simulink library "optimum_ul"  (R2018a)
settings: Solver=VariableStepAuto  StartTime=0.0  StopTime=10.0  RelTol=1e-3
settings Model: Creator=mitch  LastModifiedBy=mitch

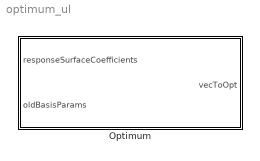
== system optimum_ul ==
  Optimum : Subsystem

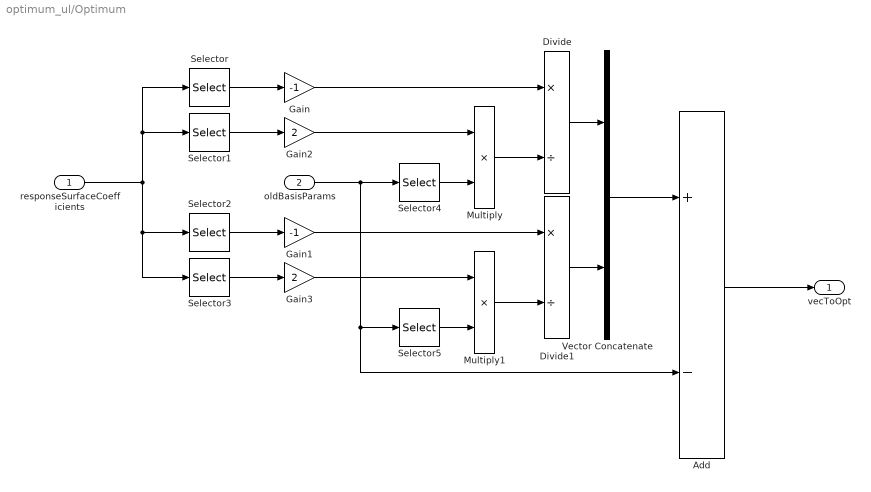
== system optimum_ul/Optimum ==
  responseSurfaceCoefficients : Inport
  oldBasisParams : Inport  Port=2
  Add : Sum  Inputs=+-
  Divide : Product  Inputs=*/
  Divide1 : Product  Inputs=*/
  Gain : Gain  Gain=-1
  Gain1 : Gain  Gain=-1
  Gain2 : Gain  Gain=2
  Gain3 : Gain  Gain=2
  Multiply : Product
  Multiply1 : Product
  Selector : Selector  InputPortWidth=5  IndexOptions=Index vector (dialog)  Indices=2  OutputSizes=1
  Selector1 : Selector  InputPortWidth=5  IndexOptions=Index vector (dialog)  Indices=3  OutputSizes=1
  Selector2 : Selector  InputPortWidth=5  IndexOptions=Index vector (dialog)  Indices=4  OutputSizes=1
  Selector3 : Selector  InputPortWidth=5  IndexOptions=Index vector (dialog)  Indices=5  OutputSizes=1
  Selector4 : Selector  InputPortWidth=2  IndexOptions=Index vector (dialog)  Indices=1  OutputSizes=1
  Selector5 : Selector  InputPortWidth=2  IndexOptions=Index vector (dialog)  Indices=2  OutputSizes=1
  Vector Concatenate : Concatenate
  vecToOpt : Outport
  wires:
  responseSurfaceCoefficients/1 -> Selector/1, Selector1/1, Selector3/1, Selector2/1
  Selector/1 -> Gain/1
  Gain/1 -> Divide/1
  Selector1/1 -> Gain2/1
  Gain2/1 -> Multiply/1
  Multiply/1 -> Divide/2
  Divide/1 -> Vector Concatenate/1
  Divide1/1 -> Vector Concatenate/2
  Selector4/1 -> Multiply/2
  oldBasisParams/1 -> Selector5/1, Add/2, Selector4/1
  Selector3/1 -> Gain3/1
  Gain1/1 -> Divide1/1
  Selector2/1 -> Gain1/1
  Multiply1/1 -> Divide1/2
  Selector5/1 -> Multiply1/2
  Gain3/1 -> Multiply1/1
  Vector Concatenate/1 -> Add/1
  Add/1 -> vecToOpt/1
